simulink model "ex2model"  (R2021a)
settings: Solver=VariableStepAuto  StartTime=0.0  StopTime=10.0  RelTol=1e-3
values from neighbouring files (symbols this model uses):
  a21 = 1/(2*m)*x30^2*FemP1/FemP2*exp(-x10/FemP2)    [ex2.m]
  a23 = -1/(m)*x30*FemP1/FemP2*exp(-x10/FemP2)    [ex2.m]
  a31 = 1/f1*exp(x10/f2)*(ki*u10+ci-x30)    [ex2.m]
  a33 = -f2/f1*exp(x10/f2)    [ex2.m]
  b31 = ki*f2/f1*exp(x10/f2)    [ex2.m]
  g = 9.81    [ex2.m]
  xd = d-bd    (= 0.0192)    [ex2.m]
settings Model: Creator=AgraWoodAdmin  LastModifiedBy=AgraWoodAdmin

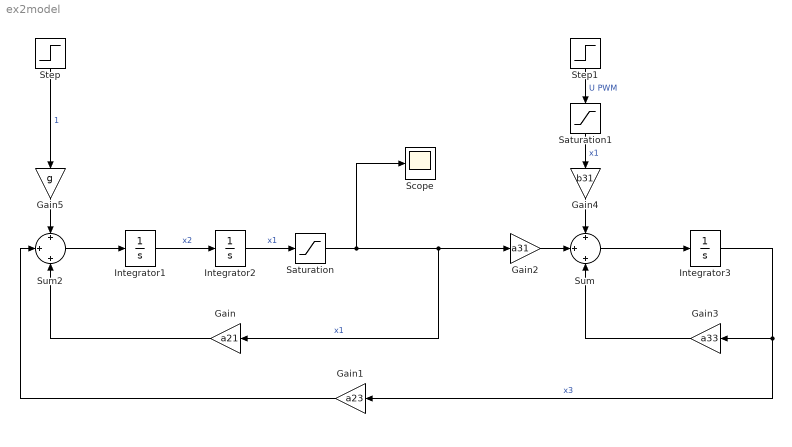
== system ex2model ==
  Gain : Gain  Gain=a21
  Gain1 : Gain  Gain=a23
  Gain2 : Gain  Gain=a31
  Gain3 : Gain  Gain=a33
  Gain4 : Gain  Gain=b31
  Gain5 : Gain  Gain=g
  Integrator1 : Integrator
  Integrator2 : Integrator
  Integrator3 : Integrator
  Saturation : Saturate  UpperLimit=xd  LowerLimit=0
  Saturation1 : Saturate  UpperLimit=1  LowerLimit=0
  Scope : Scope
  Step : Step  Time=10  SampleTime=0
  Step1 : Step  Time=10  After=10  SampleTime=0
  Sum : Sum  Inputs=+|+|+
  Sum2 : Sum  Inputs=+|+|+
  wires:
  Sum2/1 -> Integrator1/1
  Sum/1 -> Integrator3/1
  Saturation/1 -> Scope/1, Gain2/1, Gain/1  "x1"
  Integrator1/1 -> Integrator2/1  "x2"
  Integrator3/1 -> Gain3/1, Gain1/1  "x3"
  Gain/1 -> Sum2/3
  Gain1/1 -> Sum2/2
  Gain2/1 -> Sum/2
  Gain3/1 -> Sum/3
  Step1/1 -> Saturation1/1  "U PWM"
  Gain4/1 -> Sum/1
  Gain5/1 -> Sum2/1
  Step/1 -> Gain5/1  "1"
  Integrator2/1 -> Saturation/1  "x1"
  Saturation1/1 -> Gain4/1  "x1"
